simulink model "PredictiveSim"  (R2022a)
settings: Solver=FixedStepAuto  StartTime=0.0  StopTime=801  RelTol=1e-3
libraries: PredictionBlock x1
settings Model: Creator=Alia  LastModifiedBy=Skander
settings SolverCC: AlgebraicLoopSolver=TrustRegion
settings DebuggingCC: UnconnectedInputMsg=warning  UnconnectedOutputMsg=warning  UnconnectedLineMsg=warning  SFMachineParentedDataDiag=warning
settings RTWCC: DLArmComputeVersion=19.05

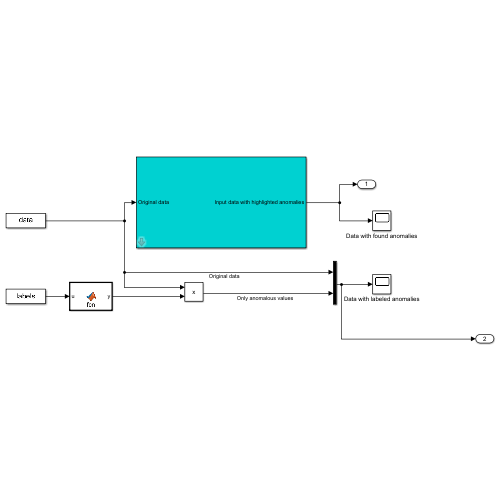
[thumbnail: Simulink's stored preview of the top-level diagram]
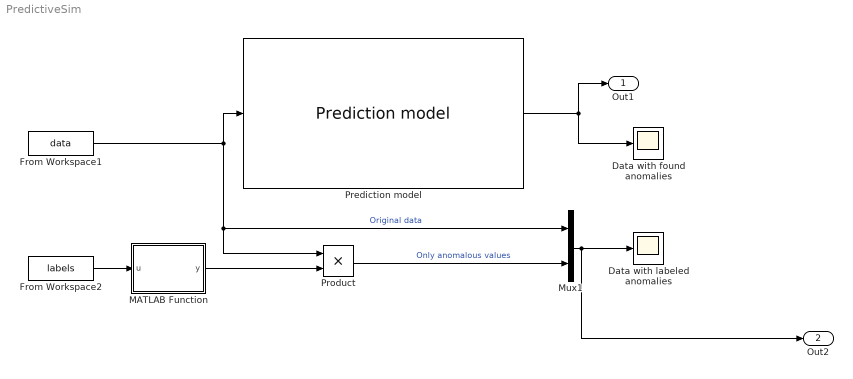
== system PredictiveSim ==
  Data with found anomalies : Scope
  Data with labeled anomalies : Scope
  From Workspace1 : FromWorkspace  VariableName=data
  From Workspace2 : FromWorkspace  VariableName=labels
  MATLAB Function : MATLAB Function  TreatAsAtomicUnit=on
  Mux1 : Mux  Inputs=2
  Prediction model : PredictionBlock/Prediction model  BufferLength=40  NetworkFilePath=C:\Users\Skander\MATLAB\Projects\TSAD2 - Copie\Exported_Models_Sim\F-4\10-31-2022\MLP_1.mat
  Product : Product
  Out1 : Outport
  Out2 : Outport  Port=2
  wires:
  Product/1 -> Mux1/2  "Only anomalous values"
  Mux1/1 -> Data with labeled anomalies/1, Out2/1
  From Workspace1/1 -> Product/1, Mux1/1, Prediction model/1  "Original data"
  MATLAB Function/1(y) -> Product/2
  From Workspace2/1 -> MATLAB Function/1(u)
  Prediction model/1 -> Out1/1, Data with found anomalies/1

== matlab function PredictiveSim/MATLAB Function ==
  data: u input; y output
function y = fcn(u)
y = NaN;
if u == 1
    y = 1;
end
